simulink model "Autoalign_system"  (R2016b)
settings: Solver=FixedStepAuto  StartTime=0.0  StopTime=inf  RelTol=1e-3  EnableMultiTasking=on
libraries: arduinolib x9
settings Model: SimulationMode=external  ExtModeEnableFloating=off  ExtModeTrigDuration=2  TunableVars=on,read_time,center_x,center_y,loops,delay,diameter  TunableVarsStorageClass=Auto,Auto,Auto,Auto,Auto,Auto,Auto  TunableVarsTypeQualifier=,,,,,,  Creator=Gebruiker  LastModifiedBy=Gebruiker
settings OptimizationCC: MaxStackSize=64
settings DebuggingCC: ParameterTunabilityLossMsg=error  AssertControl=DisableAll
settings HardwareCC: ProdBitPerInt=16  ProdBitPerPointer=16  ProdBitPerSizeT=16  ProdBitPerPtrDiffT=16  ProdLargestAtomicFloat=None  ProdWordSize=8  ProdHWDeviceType=Atmel->AVR
settings ModelReferenceCC: CheckModelReferenceTargetMessage=warning
settings RTWCC: SystemTargetFile=ert.tlc  HardwareBoard=Arduino Mega 2560  TLCOptions=-aInlineSetEventsForThisBaseRateFcn=TLC_FALSE -aSuppressMultiTaskScheduler=TLC_FALSE -aRateBasedStepFcn=1  TemplateMakefile=ert_default_tmf  Description=Embedded Coder  GenerateReport=on  Toolchain=Arduino AVR  BuildConfiguration=Faster Runs  IncludeHyperlinkInReport=on  GenerateTraceInfo=on  GenerateTraceReport=on  GenerateTraceReportSl=on  GenerateTraceReportSf=on  GenerateTraceReportEml=on
settings CodeAppCC: OperatorAnnotations=on  SimulinkDataObjDesc=on  SFDataObjDesc=on  MATLABFcnDesc=on  InsertBlockDesc=on  MATLABSourceComments=on
settings ERTTargetCC: TargetLangStandard=C99 (ISO)  SupportContinuousTime=on  SupportVariableSizeSignals=on  ExtModeMexArgs="127.0.0.1  17725 30"  RootIOFormat=Structure reference

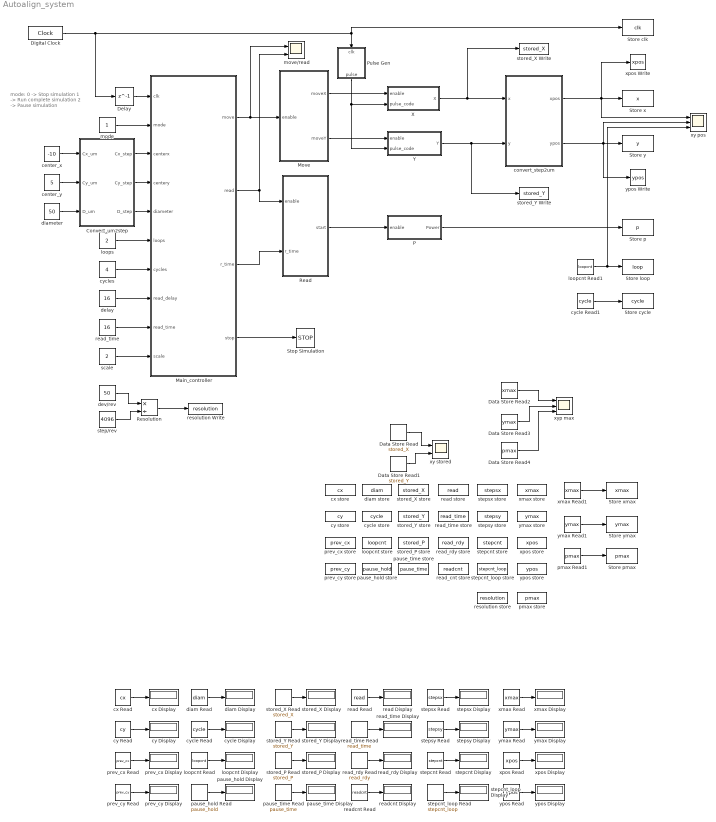
== system Autoalign_system ==
  note: mode:
      | 0 -> Stop simulation
      | 1 -> Run complete simulation
      | 2 -> Pause simulation
  Convert_um2step : MATLAB Function  TreatAsAtomicUnit=on
  Data Store Read : DataStoreRead  DataStoreName=stored_X
  Data Store Read1 : DataStoreRead  DataStoreName=stored_Y
  Data Store Read2 : DataStoreRead  DataStoreName=xmax
  Data Store Read3 : DataStoreRead  DataStoreName=ymax
  Data Store Read4 : DataStoreRead  DataStoreName=pmax
  Delay : Delay  DelayLength=1
  Digital Clock : DigitalClock  SampleTime=.00125
  Main_controller : MATLAB Function  TreatAsAtomicUnit=on
  Move : MATLAB Function  TreatAsAtomicUnit=on
  P : Subsystem  Tag=p_block
  Pulse Gen : Subsystem  Tag=t_block
  Read : MATLAB Function  TreatAsAtomicUnit=on
  Resolution : Product  Inputs=*/
  Stop Simulation : Stop
  Store clk : ToWorkspace  VariableName=clk  SampleTime=-1
      settings: PauseFcn=setappdata(0,'t_data',clk);  StopFcn=setappdata(0,'t_data',clk);
  Store cycle : ToWorkspace  VariableName=cycle  SampleTime=-1
      settings: PauseFcn=setappdata(0,'cyclenr',cycle);  StopFcn=setappdata(0,'cyclenr',cycle);
  Store loop : ToWorkspace  VariableName=loop  SampleTime=-1
      settings: PauseFcn=setappdata(0,'loopnr',loop);  StopFcn=setappdata(0,'loopnr',loop);
  Store p : ToWorkspace  VariableName=p  SampleTime=-1
      settings: PauseFcn=setappdata(0,'p_data',p);  StopFcn=setappdata(0,'p_data',p);
  Store pmax : ToWorkspace  VariableName=pmax  SampleTime=-1
      settings: PauseFcn=setappdata(0,'pmax',pmax);  StopFcn=setappdata(0,'pmax',pmax);
  Store x : ToWorkspace  VariableName=x  SampleTime=-1
      settings: PauseFcn=setappdata(0,'x_data',x);  StopFcn=setappdata(0,'x_data',x);
  Store xmax : ToWorkspace  VariableName=xmax  SampleTime=-1
      settings: PauseFcn=setappdata(0,'xmax',xmax);  StopFcn=setappdata(0,'xmax',xmax);
  Store y : ToWorkspace  VariableName=y  SampleTime=-1
      settings: PauseFcn=setappdata(0,'y_data',y);  StopFcn=setappdata(0,'y_data',y);
  Store ymax : ToWorkspace  VariableName=ymax  SampleTime=-1
      settings: PauseFcn=setappdata(0,'ymax',ymax);  StopFcn=setappdata(0,'ymax',ymax);
  X : Subsystem  Tag=y_block
  Y : Subsystem  Tag=y_block
  center_x : Constant  Value=-10
  center_y : Constant  Value=5
  convert_step2um : MATLAB Function  TreatAsAtomicUnit=on
  cx Display : Display
  cx store : DataStoreMemory  DataStoreName=cx  ReadBeforeWriteMsg=warning  WriteAfterWriteMsg=warning  WriteAfterReadMsg=warning  ShowAdditionalParam=off  OutDataTypeStr=double
  cx Read : DataStoreRead  DataStoreName=cx
  cy Display : Display
  cy store : DataStoreMemory  DataStoreName=cy  ReadBeforeWriteMsg=warning  WriteAfterWriteMsg=warning  WriteAfterReadMsg=warning  ShowAdditionalParam=off  OutDataTypeStr=double
  cy Read : DataStoreRead  DataStoreName=cy
  cycle Display : Display
  cycle Read : DataStoreRead  DataStoreName=cycle
  cycle Read1 : DataStoreRead  DataStoreName=cycle
  cycle store : DataStoreMemory  DataStoreName=cycle  ReadBeforeWriteMsg=warning  WriteAfterWriteMsg=warning  WriteAfterReadMsg=warning  InitialValue=1  ShowAdditionalParam=off  OutDataTypeStr=double
  cycles : Constant  Value=4
  delay : Constant  Value=16
  dev/rev : Constant  Value=50
  diam Display : Display
  diam Read : DataStoreRead  DataStoreName=diam
  diam store : DataStoreMemory  DataStoreName=diam  ReadBeforeWriteMsg=warning  WriteAfterWriteMsg=warning  WriteAfterReadMsg=warning  InitialValue=50  ShowAdditionalParam=off  OutDataTypeStr=double
  diameter : Constant  Value=50
  loopcnt Display : Display
  loopcnt Read : DataStoreRead  DataStoreName=loopcnt
  loopcnt Read1 : DataStoreRead  DataStoreName=loopcnt
  loopcnt store : DataStoreMemory  DataStoreName=loopcnt  ReadBeforeWriteMsg=warning  WriteAfterWriteMsg=warning  WriteAfterReadMsg=warning  InitialValue=1  ShowAdditionalParam=off  OutDataTypeStr=double
  loops : Constant  Value=2
  mode : Constant
  move/read : Scope  NumInputPorts=2
  pause_hold Display : Display
  pause_hold Read : DataStoreRead  DataStoreName=pause_hold
  pause_hold store : DataStoreMemory  DataStoreName=pause_hold  ReadBeforeWriteMsg=warning  WriteAfterWriteMsg=warning  WriteAfterReadMsg=warning  ShowAdditionalParam=off  OutDataTypeStr=double
  pause_time Display : Display
  pause_time Read : DataStoreRead  DataStoreName=pause_time
  pause_time store : DataStoreMemory  DataStoreName=pause_time  ReadBeforeWriteMsg=warning  WriteAfterWriteMsg=warning  WriteAfterReadMsg=warning  ShowAdditionalParam=off  OutDataTypeStr=double
  pmax Read1 : DataStoreRead  DataStoreName=pmax
  pmax store : DataStoreMemory  DataStoreName=pmax  ReadBeforeWriteMsg=warning  WriteAfterWriteMsg=warning  WriteAfterReadMsg=warning  ShowAdditionalParam=off  OutDataTypeStr=double
  prev_cx Display : Display
  prev_cx Read : DataStoreRead  DataStoreName=prev_cx
  prev_cx store : DataStoreMemory  DataStoreName=prev_cx  ReadBeforeWriteMsg=warning  WriteAfterWriteMsg=warning  WriteAfterReadMsg=warning  ShowAdditionalParam=off  OutDataTypeStr=double
  prev_cy Display : Display
  prev_cy Read : DataStoreRead  DataStoreName=prev_cy
  prev_cy store : DataStoreMemory  DataStoreName=prev_cy  ReadBeforeWriteMsg=warning  WriteAfterWriteMsg=warning  WriteAfterReadMsg=warning  ShowAdditionalParam=off  OutDataTypeStr=double
  read Display : Display
  read Read : DataStoreRead  DataStoreName=read
  read store : DataStoreMemory  DataStoreName=read  ReadBeforeWriteMsg=warning  WriteAfterWriteMsg=warning  WriteAfterReadMsg=warning  ShowAdditionalParam=off  OutDataTypeStr=double
  read_cnt store : DataStoreMemory  DataStoreName=readcnt  ReadBeforeWriteMsg=warning  WriteAfterWriteMsg=warning  WriteAfterReadMsg=warning  ShowAdditionalParam=off  OutDataTypeStr=double
  read_rdy Display : Display
  read_rdy Read : DataStoreRead  DataStoreName=read_rdy
  read_rdy store : DataStoreMemory  DataStoreName=read_rdy  ReadBeforeWriteMsg=warning  WriteAfterWriteMsg=warning  WriteAfterReadMsg=warning  ShowAdditionalParam=off  OutDataTypeStr=double
  read_time : Constant  Value=16
  read_time Display : Display
  read_time Read : DataStoreRead  DataStoreName=read_time
  read_time store : DataStoreMemory  DataStoreName=read_time  ReadBeforeWriteMsg=warning  WriteAfterWriteMsg=warning  WriteAfterReadMsg=warning  ShowAdditionalParam=off  OutDataTypeStr=double
  readcnt Display : Display
  readcnt Read : DataStoreRead  DataStoreName=readcnt
  resolution Write : DataStoreWrite  DataStoreName=resolution
  resolution store : DataStoreMemory  DataStoreName=resolution  ReadBeforeWriteMsg=warning  WriteAfterWriteMsg=warning  WriteAfterReadMsg=warning  ShowAdditionalParam=off  OutDataTypeStr=double
  scale : Constant  Value=2
  step/rev : Constant  Value=4096
  stepcnt Display : Display
  stepcnt Read : DataStoreRead  DataStoreName=stepcnt
  stepcnt store : DataStoreMemory  DataStoreName=stepcnt  ReadBeforeWriteMsg=warning  WriteAfterWriteMsg=warning  WriteAfterReadMsg=warning  ShowAdditionalParam=off  OutDataTypeStr=double
  stepcnt_loop Display : Display
  stepcnt_loop Read : DataStoreRead  DataStoreName=stepcnt_loop
  stepcnt_loop store : DataStoreMemory  DataStoreName=stepcnt_loop  ReadBeforeWriteMsg=warning  WriteAfterWriteMsg=warning  WriteAfterReadMsg=warning  ShowAdditionalParam=off  OutDataTypeStr=double
  stepsx Display : Display
  stepsx Read : DataStoreRead  DataStoreName=stepsx
  stepsx store : DataStoreMemory  DataStoreName=stepsx  ReadBeforeWriteMsg=warning  WriteAfterWriteMsg=warning  WriteAfterReadMsg=warning  ShowAdditionalParam=off  OutDataTypeStr=double
  stepsy Display : Display
  stepsy Read : DataStoreRead  DataStoreName=stepsy
  stepsy store : DataStoreMemory  DataStoreName=stepsy  ReadBeforeWriteMsg=warning  WriteAfterWriteMsg=warning  WriteAfterReadMsg=warning  ShowAdditionalParam=off  OutDataTypeStr=double
  stored_P Display : Display
  stored_P Read : DataStoreRead  DataStoreName=stored_P
  stored_P store : DataStoreMemory  DataStoreName=stored_P  ReadBeforeWriteMsg=warning  WriteAfterWriteMsg=warning  WriteAfterReadMsg=warning  ShowAdditionalParam=off  OutDataTypeStr=double
  stored_X Display : Display
  stored_X Read : DataStoreRead  DataStoreName=stored_X
  stored_X Write : DataStoreWrite  DataStoreName=stored_X
  stored_X store : DataStoreMemory  DataStoreName=stored_X  ReadBeforeWriteMsg=warning  WriteAfterWriteMsg=warning  WriteAfterReadMsg=warning  ShowAdditionalParam=off  OutDataTypeStr=double
  stored_Y Display : Display
  stored_Y Read : DataStoreRead  DataStoreName=stored_Y
  stored_Y Write : DataStoreWrite  DataStoreName=stored_Y
  stored_Y store : DataStoreMemory  DataStoreName=stored_Y  ReadBeforeWriteMsg=warning  WriteAfterWriteMsg=warning  WriteAfterReadMsg=warning  ShowAdditionalParam=off  OutDataTypeStr=double
  xmax Display : Display
  xmax Read : DataStoreRead  DataStoreName=xmax
  xmax Read1 : DataStoreRead  DataStoreName=xmax
  xmax store : DataStoreMemory  DataStoreName=xmax  ReadBeforeWriteMsg=warning  WriteAfterWriteMsg=warning  WriteAfterReadMsg=warning  ShowAdditionalParam=off  OutDataTypeStr=double
  xpos Display : Display
  xpos Read : DataStoreRead  DataStoreName=xpos
  xpos store : DataStoreMemory  DataStoreName=xpos  ReadBeforeWriteMsg=warning  WriteAfterWriteMsg=warning  WriteAfterReadMsg=warning  ShowAdditionalParam=off  OutDataTypeStr=double
  xpos Write : DataStoreWrite  DataStoreName=xpos
  xy pos : Scope  NumInputPorts=3
  xy stored : Scope  NumInputPorts=2
  xyp max : Scope  NumInputPorts=3
  ymax Display : Display
  ymax Read : DataStoreRead  DataStoreName=ymax
  ymax Read1 : DataStoreRead  DataStoreName=ymax
  ymax store : DataStoreMemory  DataStoreName=ymax  ReadBeforeWriteMsg=warning  WriteAfterWriteMsg=warning  WriteAfterReadMsg=warning  ShowAdditionalParam=off  OutDataTypeStr=double
  ypos Display : Display
  ypos Read : DataStoreRead  DataStoreName=ypos
  ypos store : DataStoreMemory  DataStoreName=ypos  ReadBeforeWriteMsg=warning  WriteAfterWriteMsg=warning  WriteAfterReadMsg=warning  ShowAdditionalParam=off  OutDataTypeStr=double
  ypos Write : DataStoreWrite  DataStoreName=ypos
  wires:
  Read/1(start) -> P/1(enable)
  Move/1(moveX) -> X/1(enable)
  Move/2(moveY) -> Y/1(enable)
  Pulse Gen/1(pulse) -> Y/2(pulse_code), X/2(pulse_code)
  Digital Clock/1 -> Delay/1, Store clk/1, Pulse Gen/1(clk)
  dev/rev/1 -> Resolution/1
  step/rev/1 -> Resolution/2
  cycles/1 -> Main_controller/7(cycles)
  read_time/1 -> Main_controller/9(read_time)
  Resolution/1 -> resolution Write/1
  delay/1 -> Main_controller/8(read_delay)
  Main_controller/1(move) -> move/read/1, Move/1(enable)
  Main_controller/2(read) -> Read/1(enable), move/read/2
  Main_controller/3(r_time) -> Read/2(r_time)
  Main_controller/4(stop) -> Stop Simulation/1
  P/1(Power) -> Store p/1
  loops/1 -> Main_controller/6(loops)
  convert_step2um/1(xpos) -> xy pos/1, xpos Write/1, Store x/1
  cycle Read1/1 -> Store cycle/1
  scale/1 -> Main_controller/10(scale)
  loopcnt Read1/1 -> xy pos/3, Store loop/1
  cx Read/1 -> cx Display/1
  cy Read/1 -> cy Display/1
  prev_cx Read/1 -> prev_cx Display/1
  prev_cy Read/1 -> prev_cy Display/1
  diam Read/1 -> diam Display/1
  stored_X Read/1 -> stored_X Display/1
  pause_time Read/1 -> pause_time Display/1
  stored_P Read/1 -> stored_P Display/1
  stored_Y Read/1 -> stored_Y Display/1
  cycle Read/1 -> cycle Display/1
  loopcnt Read/1 -> loopcnt Display/1
  pause_hold Read/1 -> pause_hold Display/1
  readcnt Read/1 -> readcnt Display/1
  read_rdy Read/1 -> read_rdy Display/1
  read_time Read/1 -> read_time Display/1
  read Read/1 -> read Display/1
  stepcnt_loop Read/1 -> stepcnt_loop Display/1
  stepcnt Read/1 -> stepcnt Display/1
  stepsy Read/1 -> stepsy Display/1
  stepsx Read/1 -> stepsx Display/1
  ypos Read/1 -> ypos Display/1
  xpos Read/1 -> xpos Display/1
  ymax Read/1 -> ymax Display/1
  xmax Read/1 -> xmax Display/1
  xmax Read1/1 -> Store xmax/1
  ymax Read1/1 -> Store ymax/1
  convert_step2um/2(ypos) -> xy pos/2, ypos Write/1, Store y/1
  pmax Read1/1 -> Store pmax/1
  X/1(X) -> stored_X Write/1, convert_step2um/1(x)
  Y/1(Y) -> convert_step2um/2(y), stored_Y Write/1
  mode/1 -> Main_controller/2(mode)
  Data Store Read/1 -> xy stored/1
  Data Store Read1/1 -> xy stored/2
  Data Store Read4/1 -> xyp max/3
  Data Store Read3/1 -> xyp max/2
  Data Store Read2/1 -> xyp max/1
  center_x/1 -> Convert_um2step/1(Cx_um)
  Convert_um2step/2(Cy_step) -> Main_controller/4(centery)
  Convert_um2step/1(Cx_step) -> Main_controller/3(centerx)
  Convert_um2step/3(D_step) -> Main_controller/5(diameter)
  center_y/1 -> Convert_um2step/2(Cy_um)
  diameter/1 -> Convert_um2step/3(D_um)
  Delay/1 -> Main_controller/1(clk)

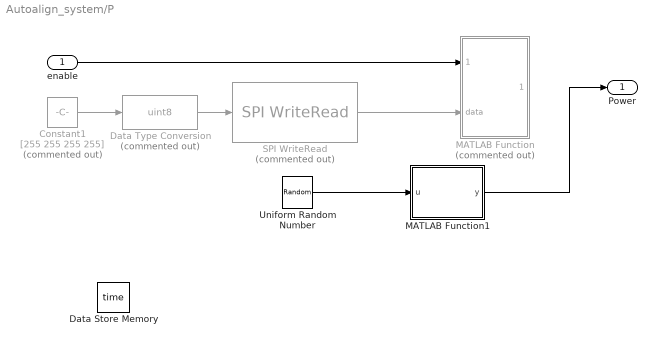
== system Autoalign_system/P ==
  enable : Inport
  Constant1 : Constant  Commented=on  Value=[255 255 255 255]
  Data Store Memory : DataStoreMemory  DataStoreName=time  ReadBeforeWriteMsg=warning  WriteAfterWriteMsg=warning  WriteAfterReadMsg=warning  ShowAdditionalParam=off  OutDataTypeStr=double
  Data Type Conversion : DataTypeConversion  Commented=on  OutDataTypeStr=uint8
  MATLAB Function : MATLAB Function  Commented=on  TreatAsAtomicUnit=on
  MATLAB Function1 : MATLAB Function  TreatAsAtomicUnit=on
  SPI WriteRead : arduinolib/SPI WriteRead  Commented=on  slaveSelectPin_=44  blockPlatform=arduino
  Uniform Random Number : UniformRandomNumber  Minimum=0  Maximum=3  Seed=10000
  Power : Outport
  wires:
  Constant1/1 -> Data Type Conversion/1
  Data Type Conversion/1 -> SPI WriteRead/1
  enable/1 -> MATLAB Function/1(enable)
  SPI WriteRead/1 -> MATLAB Function/2(data)
  Uniform Random Number/1 -> MATLAB Function1/1(u)
  MATLAB Function1/1(y) -> Power/1

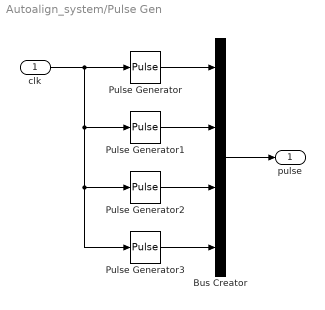
== system Autoalign_system/Pulse Gen ==
  clk : Inport
  Bus Creator : BusCreator  Inputs=4
  Pulse Generator : DiscretePulseGenerator  TimeSource=Use external signal  Period=8  PulseWidth=3
  Pulse Generator1 : DiscretePulseGenerator  TimeSource=Use external signal  Period=8  PulseWidth=3  PhaseDelay=2
  Pulse Generator2 : DiscretePulseGenerator  TimeSource=Use external signal  Period=8  PulseWidth=3  PhaseDelay=4
  Pulse Generator3 : DiscretePulseGenerator  TimeSource=Use external signal  Period=8  PulseWidth=3  PhaseDelay=6
  pulse : Outport
  wires:
  clk/1 -> Pulse Generator1/1, Pulse Generator2/1, Pulse Generator3/1, Pulse Generator/1
  Pulse Generator3/1 -> Bus Creator/4
  Pulse Generator1/1 -> Bus Creator/2
  Pulse Generator/1 -> Bus Creator/1
  Bus Creator/1 -> pulse/1
  Pulse Generator2/1 -> Bus Creator/3

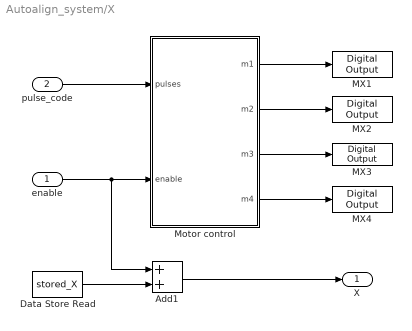
== system Autoalign_system/X ==
  enable : Inport
  pulse_code : Inport  Port=2
  Add1 : Sum
  Data Store Read : DataStoreRead  DataStoreName=stored_X
  MX1 : arduinolib/Digital Output  pinNumber=2  blockPlatform=arduino
  MX2 : arduinolib/Digital Output  pinNumber=3  blockPlatform=arduino
  MX3 : arduinolib/Digital Output  pinNumber=4  blockPlatform=arduino
  MX4 : arduinolib/Digital Output  pinNumber=5  blockPlatform=arduino
  Motor control : MATLAB Function  TreatAsAtomicUnit=on
  X : Outport
  wires:
  pulse_code/1 -> Motor control/1(pulses)
  Motor control/4(m4) -> MX4/1
  Motor control/3(m3) -> MX3/1
  Motor control/2(m2) -> MX2/1
  Motor control/1(m1) -> MX1/1
  enable/1 -> Add1/1, Motor control/2(enable)
  Add1/1 -> X/1
  Data Store Read/1 -> Add1/2

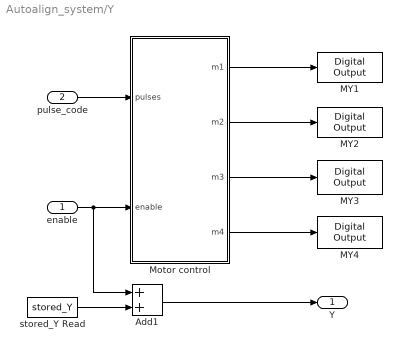
== system Autoalign_system/Y ==
  enable : Inport
  pulse_code : Inport  Port=2
  Add1 : Sum
  MY1 : arduinolib/Digital Output  pinNumber=8  blockPlatform=arduino
  MY2 : arduinolib/Digital Output  pinNumber=9  blockPlatform=arduino
  MY3 : arduinolib/Digital Output  pinNumber=10  blockPlatform=arduino
  MY4 : arduinolib/Digital Output  pinNumber=11  blockPlatform=arduino
  Motor control : MATLAB Function  TreatAsAtomicUnit=on
  stored_Y Read : DataStoreRead  DataStoreName=stored_Y
  Y : Outport
  wires:
  pulse_code/1 -> Motor control/1(pulses)
  Motor control/4(m4) -> MY4/1
  Motor control/3(m3) -> MY3/1
  Motor control/2(m2) -> MY2/1
  Motor control/1(m1) -> MY1/1
  enable/1 -> Add1/1, Motor control/2(enable)
  Add1/1 -> Y/1
  stored_Y Read/1 -> Add1/2

== matlab function Autoalign_system/Read ==
  data: enable input; start output; read_rdy data_store_memory; read_time data_store_memory; r_time input
function start = READ(enable,r_time)
global read_rdy;
global read_time;
if enable==1
    if read_rdy==0
        if read_time<=r_time
            start=0;
            read_rdy=0;
            read_time=read_time+1;
        else
            start=1;
            read_rdy=1;
            read_time=0;
        end
    else
        start=0;
        read_rdy=0;
    end
else
    start=0;
    read_rdy=0;
end

== matlab function Autoalign_system/Main_controller ==
  data: move output; read output; r_time output; clk input; mode input; centerx input; centery input; diameter input; loops input; cycles input; read_delay input; read_time input; scale input; stop output; read_rdy data_store_memory; readcnt data_store_memory; cycle data_store_memory; diam data_store_memory; cx data_store_memory; cy data_store_memory; prev_cx data_store_memory; prev_cy data_store_memory; stepsx data_store_memory; stepsy data_store_memory; stepcnt data_store_memory; stepcnt_loop data_store_memory; loopcnt data_store_memory; stored_P data_store_memory; xpos data_store_memory; ypos data_store_memory; xmax data_store_memory; ymax data_store_memory; pmax data_store_memory
function [move, read, r_time, stop] = Main_controller...
    (clk, mode, centerx, centery, diameter, loops, cycles, read_delay, read_time, scale)
% read variables
global read_rdy; global readcnt;

% conditioning variables
global cycle; global diam; 
global cx; global cy; 
global prev_cx; global prev_cy;

% move variables
global stepsx; global stepsy;
global stepcnt; global stepcnt_loop;
global loopcnt;

% highest power
global stored_P; global xpos; global ypos;
global xmax; global ymax; global pmax;
% persistent storeData;

if clk==0
	% Initialization
	cycle=1; diam=diameter;
	cx=centerx; cy=centery;
	prev_cx=0; prev_cy=0;
    if cx~=prev_cx||cy~=prev_cy
        stepsx=cx-prev_cx;
        stepsy=cy-prev_cy;
        loopcnt=0;
    else
        stepsx=0;
        stepsy=0;
        loopcnt=1;
    end
	stepcnt=0; 
    stepcnt_loop=diam/(2*loops-1);
    readcnt=read_delay;
    pmax=0;
end
% connect through
r_time=read_time;

% check for read
readcnt=readcnt+1;
if readcnt>=read_delay
    % start reading data
    move=0;
    stop=0;
    if read_rdy==1
        % data is read
        read=0;
        readcnt=0;
    else
        % still reading data
        read=1;
    end
else
    % continue code
    read=0;
    if cycle<=cycles
        if mode==1 % controlled by GUI
            % run mode
            stop=0;
            if cx~=prev_cx||cy~=prev_cy
                % MOVE to new center
                if stepsx==0 && stepsy==0
                    % steps=new point - end of current search area
                    stepsx=cx-(prev_cx-0.5*diam);
                    stepsy=cy-(prev_cy-0.5*diam);
                end
                if stepcnt<=abs(stepsy)
                    if stepsy<0
                        % move in -y direction (Down)
                        move=4;
                    elseif stepsy>0 
                        % move in +y direction (Up)
                        move=2;
                    else
                        % stop in y direction
                        move=0; 
                    end
                    stepcnt=stepcnt+1;
                elseif stepcnt<=abs(stepsx)+abs(stepsy)
                    if stepsx<0 
                        % move in -x direction (Left)
                        move=3;
                    elseif stepsx>0 
                        % move in +x direction (Right)
                        move=1;
                    else
                        % stop in x direction
                        move=0; 
                    end
                    stepcnt=stepcnt+1;
                else
                    % finished move 
                    move=0;
                    stepsx=0; stepsy=0;
                    prev_cx=cx; prev_cy=cy;
                    stepcnt=0; loopcnt=1;
                    stepcnt_loop=diam/(2*loops-1);
                end
            else
                % SEARCH highest power
                if stepcnt<=stepcnt_loop
                    % move in +x direction (Right)
                    move=1;
                    stepcnt=stepcnt+1;
                elseif stepcnt<stepcnt_loop*2
                    % move in +y direction (Up)
                    move=2;
                    stepcnt=stepcnt+1;
                elseif stepcnt<stepcnt_loop*3
                    % move in -x direction (Left)
                    move=3;
                    stepcnt=stepcnt+1;
                elseif stepcnt<stepcnt_loop*4
                    % move in -y direction (Down)
                    move=4;
                    stepcnt=stepcnt+1;
                elseif loopcnt<loops
%                     if stepcnt<(diam/(2*loops-1))+stepcnt_loop*4
                    if stepcnt<diam*(8*loopcnt-3)/(2*loops-1)
                        % move to new loop (-x,-y)
                        move=5;
                        stepcnt=stepcnt+1;
                    else
                        % loop finished, move to new new loop
                        move=0;
                        stepcnt=0;
                        loopcnt=loopcnt+1;
                        stepcnt_loop=diam*(loopcnt-0.5)/(loops-0.5);
                    end
                else
                    % cycle finished
                    move=0;
                    stepcnt=0; loopcnt=1;
                    cx=xmax; cy=ymax;
                    diam=diam/scale;
                    cycle=cycle+1;
                    stepcnt_loop=diam/(2*loops-1);
                    pmax=0;
                end
            end
        elseif mode==2 % paused
            move=0;
            stop=0;
        else % unknown / stop mode
            move=0;
            stop=0;
        end
        
        % find highest power
        if stored_P>pmax
            xmax=xpos;
            ymax=ypos;
            pmax=stored_P;
        end
    else
        % cycles finished, stopping simulation
        move=0;
        stop=1;
    end
end

== matlab function Autoalign_system/P/MATLAB Function ==
  data: enable input; power output; data input; stored_P data_store_memory
function power = CALCP(enable, data)
% variable declaration
global stored_P;

% main code
if enable==1
    % calculate new power
    powbi1=[fliplr(de2bi(data(1,1),8)) fliplr(de2bi(data(1,2),8)) fliplr(de2bi(data(1,3),8)) fliplr(de2bi(data(1,4),8))];
    pow0=bi2de(fliplr(powbi1(1,4:32)));
    pow1=double(pow0)./167772150 - 0.0015;
    stored_P=double(pow1);
end
% update power
power=stored_P;

== matlab function Autoalign_system/Move ==
  data: enable input; moveX output; moveY output
function [moveX,moveY] = MOVE(enable)
switch enable
    case 1
        moveX=1;
        moveY=0;
    case 2
        moveX=0;
        moveY=1;
    case 3
        moveX=-1;
        moveY=0;
    case 4
        moveX=0;
        moveY=-1;
    case 5
        moveX=-1;
        moveY=-1;
    otherwise
        moveX=0;
        moveY=0;
end

== matlab function Autoalign_system/X/Motor control ==
  data: pulses input; enable input; m1 output; m2 output; m3 output; m4 output
function [m1,m2,m3,m4] = MOTOR(pulses,enable)
switch enable
    case 1
        m1=pulses(1);
        m2=pulses(2);
        m3=pulses(3);
        m4=pulses(4);
    case -1
        m1=pulses(4);
        m2=pulses(3);
        m3=pulses(2);
        m4=pulses(1);
    otherwise
        m1=0;
        m2=0;
        m3=0;
        m4=0;
end

== matlab function Autoalign_system/Y/Motor control ==
  data: pulses input; enable input; m1 output; m2 output; m3 output; m4 output
function [m1,m2,m3,m4] = MOTOR(pulses,enable)
switch enable
    case 1
        m1=pulses(1);
        m2=pulses(2);
        m3=pulses(3);
        m4=pulses(4);
    case -1
        m1=pulses(4);
        m2=pulses(3);
        m3=pulses(2);
        m4=pulses(1);
    otherwise
        m1=0;
        m2=0;
        m3=0;
        m4=0;
end

== matlab function Autoalign_system/convert_step2um ==
  data: x input; y input; xpos output; ypos output; resolution data_store_memory
function [xpos,ypos] = step2um(x, y)
global resolution;
xpos=x*resolution;
ypos=y*resolution;
% function [xpos, ypos] = fcn(x, y, diameter, loops, centerx, centery, mode)
% if mode<=1
%     xpos=x/resolution;
%     ypos=y/resolution;
% else
%     xpos=x*resolution+(centerx-diameter/(4*loops-1));
%     ypos=y*resolution+(centery-diameter/(4*loops-1));
% end

== matlab function Autoalign_system/Convert_um2step ==
  data: Cx_um input; Cx_step output; Cy_um input; D_um input; Cy_step output; D_step output; resolution data_store_memory
function [Cx_step, Cy_step, D_step] = um2step(Cx_um, Cy_um, D_um)
global resolution;

Cx_step=Cx_um/resolution;
Cy_step=Cy_um/resolution;
D_step=D_um/resolution;

== matlab function Autoalign_system/P/MATLAB Function1 ==
  data: u input; y output; stored_P data_store_memory; time data_store_memory
function y = fcn(u)
global stored_P;
global time;
if time>200
    time=0;
    stored_P=u;
else
    time=time+1;
end
y = stored_P;
